simulink model "two_async_clks"  (Simulink 7.0)
settings: Solver=ode45  StartTime=0.0  StopTime=1500  RelTol=1e-3
libraries: xbsIndex_r4 x19, xbsCopyrightNotice_r4 x1
settings Model: Creator=alexc  LastModifiedBy=juttu
settings DataIOCC: SignalLoggingName=sigsOut
settings OptimizationCC: InlineInvariantSignals=on
settings DebuggingCC: SaveWithParameterizedLinksMsg=none  SignalResolutionControl=TryResolveAllWithWarning  SolverPrmCheckMsg=none  MultiTaskDSMMsg=warning  MultiTaskCondExecSysMsg=none  StrictBusMsg=None
settings HardwareCC: TargetUnknown=on
settings RTWCC: IncludeERTFirstTime=on
settings GRTTargetCC: TargetFcnLib=ansi_tfl_tmw.mat

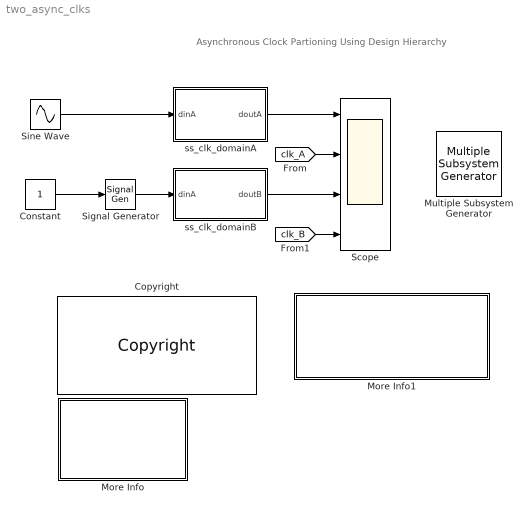
== system two_async_clks ==
  note: Asynchronous Clock Partioning
      | Using Design Hierarchy
  Constant : Constant  OutDataType=sfix(16)  OutScaling=2^0  SampleTime=3
  Copyright : xbsCopyrightNotice_r4/Copyright  block_type=copyright
      settings: block_version=10.1.00
      settings: infoedit=|
      | Copyright(C) 2008 by  Xilinx, Inc. All rights reserved.<br>
      | <br>
      | This file contains proprietary, confidential information of Xilinx, Inc., is distributed under license
      | from Xilinx, Inc., and may be used, copied and/or disclosed only pursuant to the terms of a valid license
      | agreement with Xilinx, Inc. Xilinx hereby grants you a license to use this file solely for design,
      | simulation, implementation and creation of design files limited to Xilinx devices or technologies. Use
      | with non-Xilinx devices or technologies is expressly prohibited and immediately terminates your license
      | unless covered by a separate agreement.<br>
      | <br>
      | Xilinx is providing this design, code, or information "as-is" solely for use in developing programs and
      | solutions for Xilinx devices, with no obligation on the part of Xilinx to provide support. By providing
      | this design, code, or information as one possible implementation of this feature, application or standard,
      | Xilinx is making no representation that this implementation is free from any claims of infringement. You
      | are responsible for obtaining any rights you may require for your implementation. Xilinx expressly disclaims
      | any warranty whatsoever with respect to the adequacy of the implementation, including but not limited to any
      | warranties or representations that this implementation is free from claims of infringement, implied warranties
      | of merchantability or fitness for a particular purpose.<br>
      | <br>
      | Xilinx products are not intended for use in life support appliances, devices, or systems. Use in such
      | applications is expressly prohibited.<br>
      | <br>
      | Any modifications that are made to the Source Code are done at the user's sole risk and will be unsupported.<br>
      | <br>
      | This copyright and support notice must be retained as part of this text at all times.
      | (c) Copyright 1995-2008 Xilinx, Inc. All rights reserved.
  More Info : Subsystem
      mask Display: disp('Double click\n for\n more information.')
  More Info1 : Subsystem
      settings: OpenFcn=xlDoc('-book','sysgen','-topic','Hardware Design Using System Generator/Generating Multiple Cycle-True Islands for Distinct Clocks');
      mask Display: disp('Double click\n for System Generator\n documentation on related topics.')
  Multiple Subsystem Generator : xbsIndex_r4/Multiple Subsystem Generator  Tag=xlStitcher  block_type=msg
      settings: AttributesFormatString=Multiple Subsystem\nGenerator  infoedit=Multiple Subsystem\nGenerator  block_version=9.2.00
  Scope : Scope  NumInputPorts=4
      settings: TimeRange=1500  YMin=-5~-5~-5~-5  YMax=5~5~5~5
  Signal Generator : SignalGenerator  WaveForm=sawtooth  TimeSource=Use external signal  Frequency=(2*pi)/(256)  Units=rad/sec
  Sine Wave : Sin  Frequency=(2*pi)/(256)  SampleTime=2
  ss_clk_domainA : Subsystem
  ss_clk_domainB : Subsystem
  wires:
  Sine Wave/1 -> ss_clk_domainA/1(dinA)
  [clk_A] -> Scope/2
  [clk_B] -> Scope/4
  Signal Generator/1 -> ss_clk_domainB/1(dinA)
  ss_clk_domainA/1(doutA) -> Scope/1
  ss_clk_domainB/1(doutB) -> Scope/3
  Constant/1 -> Signal Generator/1

== system two_async_clks/More Info ==
  note: Asynchronous Clock Partioning Using Design Heirarchy
  note: Example use of hierarchy to get System Generator to netlist out a shared
      | memory interface between two cycle-true islands.  One island,
      | ss_clk_domainA, has a system sample time of 2, the other,
      | ss_clk_domainB, a system sample time of 3.  The two islands sample
      | separate input sources, and write the respective data into different halves
      | of a shared memory pair.  The two clocks may be visualized by simulating
      | the design and examining the output scope.   Use the Multiple Subsystem
      | Generator block to netlist the complete design.
      |
      | For more information, please refer to the System Generator User Guide
      | section entitled  "Generating Multiple Cycle-True Islands for Distinct Clocks."

== system two_async_clks/More Info1 ==

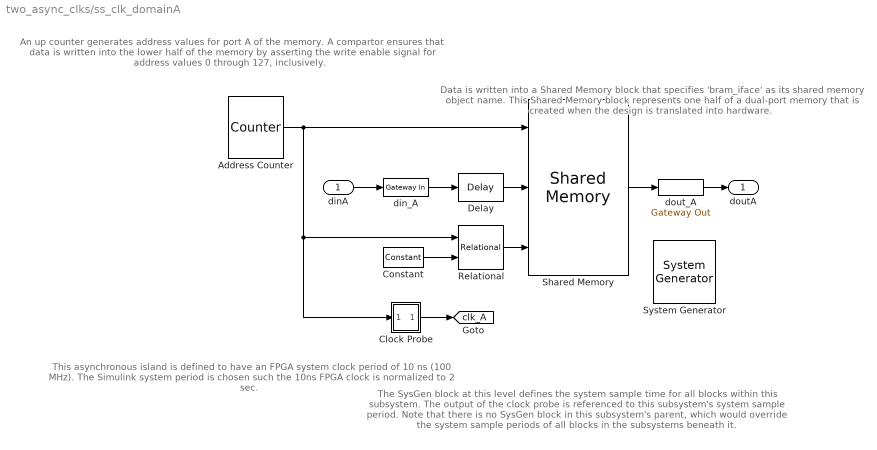
== system two_async_clks/ss_clk_domainA ==
  note: This asynchronous island is defined to have an FPGA
      | system clock period of 10 ns (100 MHz).  The Simulink
      | system period is chosen such the 10ns FPGA clock is
      | normalized to 2 sec.
  note: The SysGen block at this level defines the system
      | sample time for all blocks within this subsystem.
      | The output of the clock probe is referenced to this
      | subsystem's system sample period.  Note that
      | there is no SysGen block in this subsystem's parent,
      | which would override the system sample periods of
      | all blocks in the subsystems beneath it.
  note: An up counter generates address values for port A of the memory.  A
      | compartor ensures that data is written into the lower half of the memory
      | by asserting the write enable signal for address values 0 through 127,
      | inclusively.
  note: Data is written into a Shared Memory block that
      | specifies 'bram_iface' as its shared memory
      | object name.  This Shared Memory block
      | represents one half of a dual-port memory that
      | is created when the design is translated into
      | hardware.
  dinA : Inport  OutDataType=sfix(16)  OutScaling=2^0
  " System Generator" : xbsIndex_r4/ System Generator  Tag=genX  SystemSampleTime=-1  xilinxfamily=virtex5  part=xc5vsx50t  speed=-1  package=ff1136  synthesis_tool=XST  clock_wrapper=Clock Enables  directory=./netlist_domain_a  testbench=off  simulink_period=2  sysclk_period=10  dcm_input_clock_period=100  incr_netlist=off  trim_vbits=Everywhere in SubSystem  dbl_ovrd=According to Block Masks  core_generation=According to Block Masks  run_coregen=off  deprecated_control=off  eval_field=0  block_type=sysgen
      settings: block_version=9.2.00
  Address Counter : xbsIndex_r4/Counter  cnt_type=Free Running  cnt_to=Inf  operation=Up  start_count=0  cnt_by_val=1  arith_type=Unsigned  n_bits=8  bin_pt=0  load_pin=off  rst=off  en=off  explicit_period=off  period=2  dbl_ovrd=off  use_behavioral_HDL=off  use_rpm=off  implementation=Fabric  block_type=counter
      settings: xl_area=[0, 0, 0, 0, 0, 0, 0]  block_version=VER_STRING_GOES_HERE
  Clock Probe : Subsystem
      settings: CopyFcn=set_param(gcb, 'LinkStatus', 'none');
      mask Display: disp('CLK')
  Constant : xbsIndex_r4/Constant  arith_type=Unsigned  const=127  n_bits=7  bin_pt=0  explicit_period=off  period=1  equ=P=C  opselect=C  inp2=PCIN>>17  opr=+  inp1=P  carry=CIN  dbl_ovrd=off  block_type=constant
      settings: block_version=VER_STRING_GOES_HERE
  Delay : xbsIndex_r4/Delay  en=off  latency=1  dbl_ovrd=off  reg_retiming=off  block_type=delay
      settings: infoedit=Hardware notes: A delay line is a chain, each link of which is an SRL16 followed by a flip-flop. If register retiming is enabled, the delay line is a chain of flip-flops.  xl_area=[0, 0, 0, 0, 0, 0, 0]  block_version=VER_STRING_GOES_HERE
  Relational : xbsIndex_r4/Relational  mode=a<=b  en=off  latency=0  dbl_ovrd=off  block_type=relational
      settings: xl_area=[0, 0, 0, 0, 0, 0, 0]  block_version=VER_STRING_GOES_HERE
  Shared Memory : xbsIndex_r4/Shared Memory  shared_memory_name='bram_iface'  depth=256  ownership=Locally Owned and Initialized  initVector=0  mutex=Unprotected  mode=Read and Write  write_mode=Read After Write  time_out=0  latency=1  explicit_data_type=off  arith_type=Unsigned  n_bits=0  bin_pt=0  implementation=Block RAM  use_rpm=off  block_type=shmem
      settings: AttributesFormatString=<< %<shared_memory_name> >>  xl_area=[0, 0, 0, 0, 0, 0, 0]  block_version=VER_STRING_GOES_HERE
  din_A : xbsIndex_r4/Gateway In  arith_type="Signed  (2's comp)"  n_bits=8  bin_pt=7  quantization="Round  (unbiased: +/- Inf)"  overflow=Saturate  period=2  dbl_ovrd=off  timing_constraint=None  locs_specified=off  LOCs={}  block_type=gatewayin
      settings: infoedit="Gateway in block.  Converts inputs of type Simulink integer, double and fixed point to  Xilinx fixed point type.<P><P>Hardware notes:  In hardware these blocks become top level input ports."  xl_area=[0, 0, 0, 0, 0, 0, 0]  block_version=VER_STRING_GOES_HERE
  dout_A : xbsIndex_r4/Gateway Out  hdl_port=on  timing_constraint=None  locs_specified=off  LOCs={}  block_type=gatewayout
      settings: infoedit="Gateway out block.  Converts Xilinx fixed point inputs into ouputs of type Simulink integer, double, or fixed point.<P><P>Hardware notes:  In hardware these blocks become top level output ports or are discarded, depending on how they are configured."  xl_area=[0, 0, 0, 0, 0, 0, 0]  block_version=VER_STRING_GOES_HERE
  doutA : Outport  OutDataType=sfix(16)  OutScaling=2^0
  tag scope: clk_A=global
  wires:
  dinA/1 -> din_A/1
  Address Counter/1 -> Shared Memory/1, Relational/1, Clock Probe/1(din)
  din_A/1 -> Delay/1
  Constant/1 -> Relational/2
  Relational/1 -> Shared Memory/3
  Clock Probe/1(CLK) -> [clk_A]
  Delay/1 -> Shared Memory/2
  Shared Memory/1 -> dout_A/1
  dout_A/1 -> doutA/1

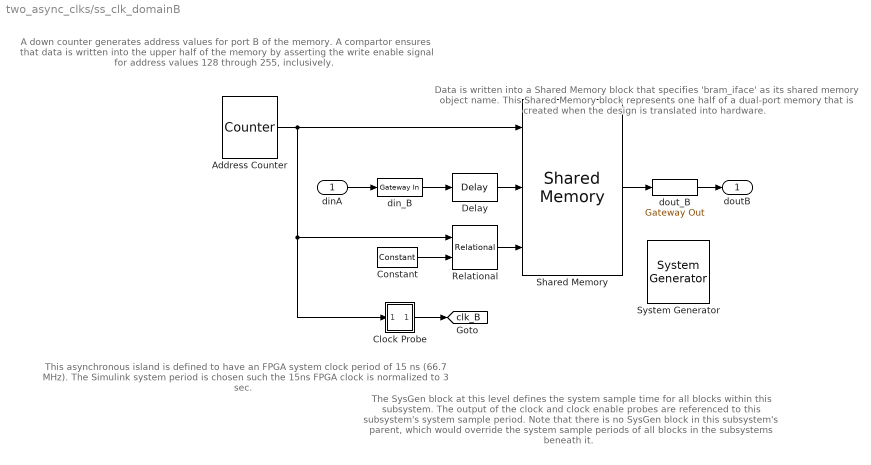
== system two_async_clks/ss_clk_domainB ==
  note: This asynchronous island is defined to have an FPGA
      | system clock period of 15 ns (66.7 MHz).  The Simulink
      | system period is chosen such the 15ns FPGA clock is
      | normalized to 3 sec.
  note: The SysGen block at this level defines the system
      | sample time for all blocks within this subsystem.
      | The output of the clock and clock enable probes are
      | referenced to this subsystem's system sample
      | period.  Note that there is no SysGen block in this
      | subsystem's parent, which would override the system
      | sample periods of all blocks in the subsystems
      | beneath it.
  note: A down counter generates address values for port B of the memory.  A
      | compartor ensures that data is written into the upper half of the memory
      | by asserting the write enable signal for address values 128 through 255,
      | inclusively.
  note: Data is written into a Shared Memory block that
      | specifies 'bram_iface' as its shared memory
      | object name.  This Shared Memory block
      | represents one half of a dual-port memory that
      | is created when the design is translated into
      | hardware.
  dinA : Inport  OutDataType=sfix(16)  OutScaling=2^0
  " System Generator" : xbsIndex_r4/ System Generator  Tag=genX  SystemSampleTime=-1  xilinxfamily=virtex5  part=xc5vsx50t  speed=-1  package=ff1136  synthesis_tool=XST  clock_wrapper=Clock Enables  directory=./netlist_domain_b  testbench=off  simulink_period=3  sysclk_period=15  dcm_input_clock_period=100  incr_netlist=off  trim_vbits=Everywhere in SubSystem  dbl_ovrd=According to Block Masks  core_generation=According to Block Masks  run_coregen=off  deprecated_control=off  eval_field=0  block_type=sysgen
      settings: block_version=9.2.00
  Address Counter : xbsIndex_r4/Counter  cnt_type=Free Running  cnt_to=Inf  operation=Down  start_count=255  cnt_by_val=1  arith_type=Unsigned  n_bits=8  bin_pt=0  load_pin=off  rst=off  en=off  explicit_period=off  period=3  dbl_ovrd=off  use_behavioral_HDL=off  use_rpm=off  implementation=Fabric  block_type=counter
      settings: xl_area=[0, 0, 0, 0, 0, 0, 0]  block_version=VER_STRING_GOES_HERE
  Clock Probe : Subsystem
      settings: CopyFcn=set_param(gcb, 'LinkStatus', 'none');
      mask Display: disp('CLK')
  Constant : xbsIndex_r4/Constant  arith_type=Unsigned  const=127  n_bits=7  bin_pt=0  explicit_period=off  period=1  equ=P=C  opselect=C  inp2=PCIN>>17  opr=+  inp1=P  carry=CIN  dbl_ovrd=off  block_type=constant
      settings: block_version=VER_STRING_GOES_HERE
  Delay : xbsIndex_r4/Delay  en=off  latency=1  dbl_ovrd=off  reg_retiming=off  block_type=delay
      settings: infoedit=Hardware notes: A delay line is a chain, each link of which is an SRL16 followed by a flip-flop. If register retiming is enabled, the delay line is a chain of flip-flops.  xl_area=[0, 0, 0, 0, 0, 0, 0]  block_version=VER_STRING_GOES_HERE
  Relational : xbsIndex_r4/Relational  mode=a>b  en=off  latency=0  dbl_ovrd=off  block_type=relational
      settings: xl_area=[0, 0, 0, 0, 0, 0, 0]  block_version=VER_STRING_GOES_HERE
  Shared Memory : xbsIndex_r4/Shared Memory  shared_memory_name='bram_iface'  depth=256  ownership=Owned and Initialized Elsewhere  initVector=0  mutex=Unprotected  mode=Read and Write  write_mode=Read After Write  time_out=0  latency=1  explicit_data_type=off  arith_type=Unsigned  n_bits=0  bin_pt=0  implementation=Block RAM  use_rpm=off  block_type=shmem
      settings: AttributesFormatString=<< %<shared_memory_name> >>  xl_area=[0, 0, 0, 0, 0, 0, 0]  block_version=VER_STRING_GOES_HERE
  din_B : xbsIndex_r4/Gateway In  arith_type="Signed  (2's comp)"  n_bits=8  bin_pt=7  quantization="Round  (unbiased: +/- Inf)"  overflow=Saturate  period=3  dbl_ovrd=off  timing_constraint=None  locs_specified=off  LOCs={}  block_type=gatewayin
      settings: infoedit="Gateway in block.  Converts inputs of type Simulink integer, double and fixed point to  Xilinx fixed point type.<P><P>Hardware notes:  In hardware these blocks become top level input ports."  xl_area=[0, 0, 0, 0, 0, 0, 0]  block_version=VER_STRING_GOES_HERE
  dout_B : xbsIndex_r4/Gateway Out  hdl_port=on  timing_constraint=None  locs_specified=off  LOCs={}  block_type=gatewayout
      settings: infoedit="Gateway out block.  Converts Xilinx fixed point inputs into ouputs of type Simulink integer, double, or fixed point.<P><P>Hardware notes:  In hardware these blocks become top level output ports or are discarded, depending on how they are configured."  xl_area=[0, 0, 0, 0, 0, 0, 0]  block_version=VER_STRING_GOES_HERE
  doutB : Outport  OutDataType=sfix(16)  OutScaling=2^0
  tag scope: clk_B=global
  wires:
  dinA/1 -> din_B/1
  Address Counter/1 -> Shared Memory/1, Clock Probe/1(din), Relational/1
  din_B/1 -> Delay/1
  Relational/1 -> Shared Memory/3
  Clock Probe/1(CLK) -> [clk_B]
  Delay/1 -> Shared Memory/2
  Shared Memory/1 -> dout_B/1
  dout_B/1 -> doutB/1
  Constant/1 -> Relational/2

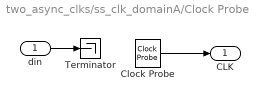
== system two_async_clks/ss_clk_domainA/Clock Probe ==
  din : Inport  OutDataType=sfix(16)  OutScaling=2^0
  Clock Probe : xbsIndex_r4/Clock Probe  SystemSampleTime=-1  block_type=clkprobe
      settings: infoedit="Clock probe.  Produces an output of type double that mirrors the hardware system clock.<P><P>Hardware notes:  This block is ignored when hardware is generated."  block_version=VER_STRING_GOES_HERE
  Terminator : Terminator
  CLK : Outport  OutDataType=sfix(16)  OutScaling=2^0
  wires:
  Clock Probe/1 -> CLK/1
  din/1 -> Terminator/1

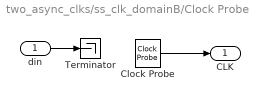
== system two_async_clks/ss_clk_domainB/Clock Probe ==
  din : Inport  OutDataType=sfix(16)  OutScaling=2^0
  Clock Probe : xbsIndex_r4/Clock Probe  SystemSampleTime=-1  block_type=clkprobe
      settings: infoedit="Clock probe.  Produces an output of type double that mirrors the hardware system clock.<P><P>Hardware notes:  This block is ignored when hardware is generated."  block_version=VER_STRING_GOES_HERE
  Terminator : Terminator
  CLK : Outport  OutDataType=sfix(16)  OutScaling=2^0
  wires:
  Clock Probe/1 -> CLK/1
  din/1 -> Terminator/1
